simulink model "TwinRotor_g1"  (Simulink 6.1)
settings: Solver=ode1  SolverMode=SingleTasking  StartTime=0.0  StopTime=500  FixedStep=0.05  RelTol=1e-3
values from neighbouring files (symbols this model uses):
  Kd_tr = 0.01    [def_pid.m]
  Ki_mr = 0.2    [def_pid.m]
  Ki_tr = 0.01    [def_pid.m]
  Kp_mr = 0.05    [def_pid.m]
  Kp_tr = 0.01    [def_pid.m]
libraries: simulink x2, RT x1
settings Model: Creator=Tomás  LastModifiedBy=Zadeh2
settings DataIOCC: SignalLoggingName=sigsOut
settings HardwareCC: TargetUnknown=on

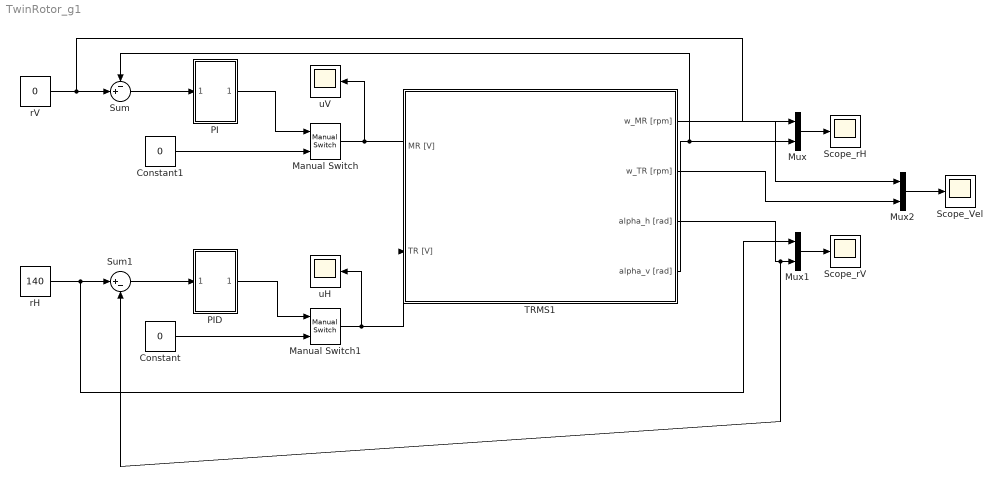
== system TwinRotor_g1 ==
  Constant : Constant  Value=0  OutDataType=fixdt(1,16,0)  OutScaling=[]
  Constant1 : Constant  Value=0  OutDataType=fixdt(1,16,0)  OutScaling=[]
  Manual Switch : simulink/Signal Routing/Manual Switch  sw=0  action=0
  Manual Switch1 : simulink/Signal Routing/Manual Switch  sw=0  action=0
  Mux : Mux  Inputs=2
  Mux1 : Mux  Inputs=2
  Mux2 : Mux  Inputs=2
  PI : Subsystem
  PID : Subsystem
  Scope_Vel : Scope
      settings: YMin=-0.125  YMax=6.125  SaveName=Velocidad  DataFormat=Array  SampleTime=-1
  Scope_rH : Scope
      settings: YMin=-0.125  YMax=6.125  SaveName=rV  DataFormat=Array  SampleTime=-1
  Scope_rV : Scope
      settings: YMin=-0.125  YMax=1.125  SaveName=rH  DataFormat=Array  SampleTime=-1
  Sum : Sum  Inputs=-+|  OutDataType=fixdt(1,16,0)  OutScaling=[]
  Sum1 : Sum  Inputs=|+-  OutDataType=fixdt(1,16,0)  OutScaling=[]
  TRMS1 : Subsystem  mask{Ts=0.05, bias_h=0, bias_v=0, max_mr=20, max_tr=15}
      mask prompts: Ts "Tiempo de Muestreo"; bias_h "bias alpha_h"; bias_v "bias alpha_v"; max_mr "voltaje MR [V]"; max_tr "voltaje TR [V]"
      mask Display:
      | image(imread('Imagenes/Copter.png'))
      | 
      | port_label('output', 1, 'w_MR [rpm]')
      | port_label('output', 2, 'w_TR [rpm]')
      | port_label('output', 3, 'alpha_h [deg]')
      | port_label('output', 4, 'alpha_v [deg]')
      | port_label('input', 1, 'MR [V]')
      | port_label('input', 2, 'TR [V]')
  rH : Constant  Value=140  OutDataType=fixdt(1,16,0)  OutScaling=[]
  rV : Constant  Value=0  OutDataType=fixdt(1,16,0)  OutScaling=[]
  uH : Scope
      settings: YMin=-1.00000  YMax=1.00000  SaveName=uH  DataFormat=Array  SampleTime=-1
  uV : Scope
      settings: YMin=-27.625  YMax=3.625  SaveName=uV  DataFormat=Array  SampleTime=-1
  wires:
  PI/1(Out1) -> Manual Switch/1
  PID/1(Out1) -> Manual Switch1/1
  Constant/1 -> Manual Switch1/2
  Constant1/1 -> Manual Switch/2
  Sum/1 -> PI/1(In1)
  Sum1/1 -> PID/1(In1)
  Manual Switch/1 -> uV/1, TRMS1/1(MR [V])
  Manual Switch1/1 -> uH/1, TRMS1/2(TR [V])
  rV/1 -> Mux/1, Sum/2
  TRMS1/4(alpha_v [rad]) -> Mux/2, Sum/1
  Mux/1 -> Scope_rH/1
  rH/1 -> Mux1/1, Sum1/1
  Mux1/1 -> Scope_rV/1
  TRMS1/3(alpha_h [rad]) -> Mux1/2, Sum1/2
  Mux2/1 -> Scope_Vel/1
  TRMS1/1(w_MR [rpm]) -> Mux2/1
  TRMS1/2(w_TR [rpm]) -> Mux2/2

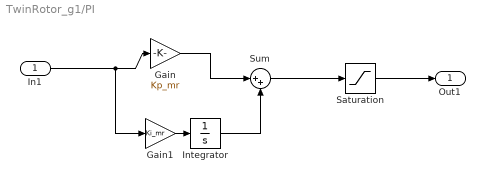
== system TwinRotor_g1/PI ==
  In1 : Inport  Port=1  LatchInput=off
  Gain : Gain  Gain=Kp_mr
  Gain1 : Gain  Gain=Ki_mr
  Integrator : Integrator
  Saturation : Saturate  UpperLimit=20  LowerLimit=0
  Sum : Sum  Inputs=|++
  Out1 : Outport
  wires:
  In1/1 -> Gain1/1, Gain/1
  Gain/1 -> Sum/1
  Integrator/1 -> Sum/2
  Gain1/1 -> Integrator/1
  Sum/1 -> Saturation/1
  Saturation/1 -> Out1/1

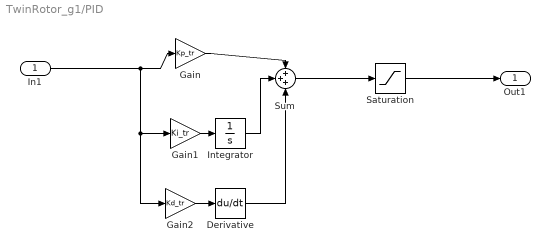
== system TwinRotor_g1/PID ==
  In1 : Inport  Port=1  LatchInput=off
  Derivative : Derivative
  Gain : Gain  Gain=Kp_tr
  Gain1 : Gain  Gain=Ki_tr
  Gain2 : Gain  Gain=Kd_tr
  Integrator : Integrator
  Saturation : Saturate  UpperLimit=5  LowerLimit=-5
  Sum : Sum  Inputs=+++
  Out1 : Outport
  wires:
  In1/1 -> Gain/1, Gain1/1, Gain2/1
  Gain/1 -> Sum/1
  Integrator/1 -> Sum/2
  Gain1/1 -> Integrator/1
  Gain2/1 -> Derivative/1
  Derivative/1 -> Sum/3
  Sum/1 -> Saturation/1
  Saturation/1 -> Out1/1

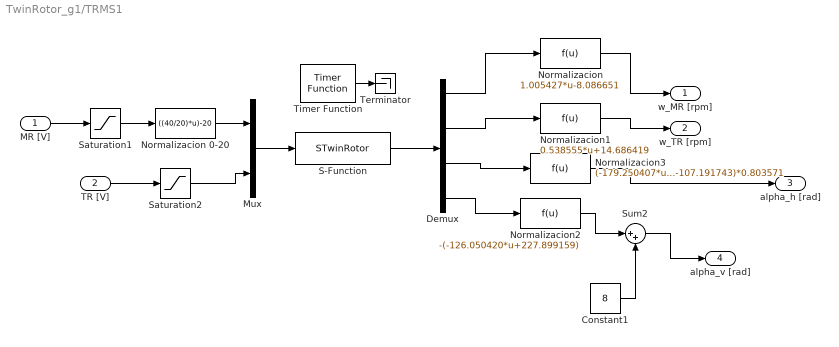
== system TwinRotor_g1/TRMS1 ==
  MR [V] : Inport  Port=1  LatchInput=off
  TR [V] : Inport  Port=2  LatchInput=off
  Constant1 : Constant  Value=8
  Demux : Demux
  Mux : Mux  Inputs=2
  Normalizacion : Fcn  Expr=1.005427*u-8.086651
  Normalizacion 0-20 : Fcn  Expr=((40/20)*u)-20
  Normalizacion1 : Fcn  Expr=0.538555*u+14.686419
  Normalizacion2 : Fcn  Expr=-(-126.050420*u+227.899159)
  Normalizacion3 : Fcn  Expr=(-179.250407*u-107.191743)*0.803571
  S-Function : S-Function  FunctionName=STwinRotor  Parameters=Ts,bias_h,bias_v,max_mr,max_tr
  Saturation1 : Saturate  UpperLimit=20  LowerLimit=0
  Saturation2 : Saturate  UpperLimit=5  LowerLimit=-5
  Sum2 : Sum  Inputs=|++
  Terminator : Terminator
  Timer Function : RT/Timer Function  Priority=827901968  step=50  priority=HIGH  ThPriority=TIME CRITICAL
  w_MR [rpm] : Outport
  w_TR [rpm] : Outport  Port=2
  alpha_h [rad] : Outport  Port=3
  alpha_v [rad] : Outport  Port=4
  wires:
  Constant1/1 -> Sum2/2
  Sum2/1 -> alpha_v [rad]/1
  Normalizacion2/1 -> Sum2/1
  Saturation2/1 -> Mux/2
  Saturation1/1 -> Normalizacion 0-20/1
  Normalizacion3/1 -> alpha_h [rad]/1
  Demux/3 -> Normalizacion3/1
  Demux/4 -> Normalizacion2/1
  Demux/2 -> Normalizacion1/1
  Normalizacion1/1 -> w_TR [rpm]/1
  Demux/1 -> Normalizacion/1
  Normalizacion/1 -> w_MR [rpm]/1
  MR [V]/1 -> Saturation1/1
  Normalizacion 0-20/1 -> Mux/1
  S-Function/1 -> Demux/1
  Mux/1 -> S-Function/1
  TR [V]/1 -> Saturation2/1
  Timer Function/1 -> Terminator/1
